simulink model "L_detector_v2"  (Simulink 7.6)
settings: Solver=FixedStepDiscrete  StartTime=0.0  StopTime=0  RelTol=1e-3
values from neighbouring files (symbols this model uses):
  Forward_Camera_Dimensions = [160 120]    [VisionConstants.m]
  Iter_Segment_Thresh = 60    [VisionConstants.m]
undefined symbols (not defined in the file or in its folder): a_range, b_range, Forward_Fov, Rec, SDTV
libraries: vipgeotforms x3, vipconversions x2, viptextngfix x1, vipanalysis x1, viptransforms x1
settings Model: Creator=Thing 1  LastModifiedBy=auvt
settings OptimizationCC: OptimizeModelRefInitCode=on
settings RTWCC: SystemTargetFile=ert.tlc  GenCodeOnly=on  TemplateMakefile=ert_default_tmf  Description=Real-Time Workshop Embedded Coder  GenerateReport=on  ProcessScript=ert_make_rtw_hook  IncludeHyperlinkInReport=on  LaunchReport=on  TargetLang=C++
settings CodeAppCC: IgnoreCustomStorageClasses=off
settings ERTTargetCC: MultiwordLength=2048  GenerateSampleERTMain=on  ERTCustomFileTemplate=example_file_process.tlc  ConvertIfToSwitch=off

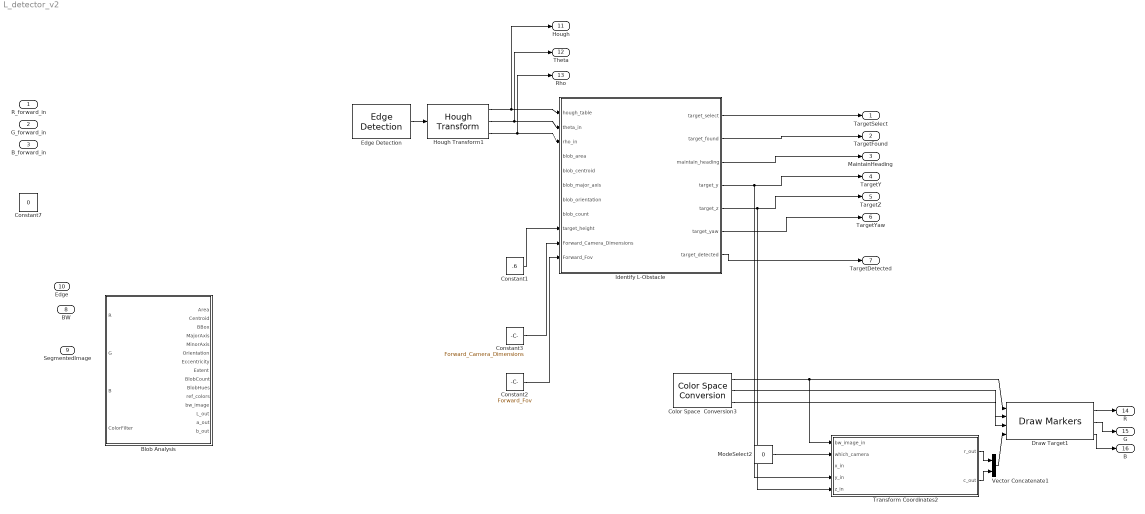
== system L_detector_v2 ==
  R_forward_in : Inport  PortDimensions=Forward_Camera_Dimensions
  G_forward_in : Inport  Port=2  PortDimensions=Forward_Camera_Dimensions
  B_forward_in : Inport  Port=3  PortDimensions=Forward_Camera_Dimensions
  Blob Analysis : Subsystem
  Color Space  Conversion3 : vipconversions/Color Space  Conversion  conversion=Obsolete  conversionActive=L*a*b* to sR'G'B'  wp_str=D50  rec=Rec. 601 (SDTV)  sys=1125/60/2:1  imagePorts=Separate color signals
  Constant1 : Constant  Value=.6  SampleTime=-1
  Constant2 : Constant  Value=Forward_Fov  SampleTime=-1
  Constant3 : Constant  Value=Forward_Camera_Dimensions  SampleTime=-1
  Constant7 : Constant  Value=0  SampleTime=-1
  Draw Target1 : viptextngfix/Draw Markers  DialogController=vipDDGCreate  DialogControllerArgs=DataTag3  shape=X-mark  size=7  fill=off  fillClrSource=Specify via dialog  display=User-specified value  intensity=200  color=[0 0 0]  opacity=0.6  viewport=Entire image  antialiasing=off  inType=Obsolete  imagePorts=Separate color signals  prodOutputMode=Binary point scaling  prodOutputWordLength=32  prodOutputFracLength=14  memoryMode=Specify word length  memoryWordLength=16  memoryFracLength=15  roundingMode=Floor  overflowMode=off
  Edge Detection : vipanalysis/Edge Detection  DialogController=vipDDGCreate  DialogControllerArgs=DataTag4  method=Sobel  outputType=Binary image  userDefinedThreshold=off  thresholdSource=Specify via dialog  threshold=20  thresholdTuning=3  edgeThinning=on  threshold_canny=[0.25 0.60]  autoPercent=70  sigma=1  roundingMode=Floor  overflowMode=off
  Hough Transform1 : viptransforms/Hough Transform  DialogController=vipDDGCreate  DialogControllerArgs=DataTag5  theta_res=pi/180  rho_res=1  out_theta_rho=on  outdtmode=double  firstCoeffMode=Binary point scaling  firstCoeffWordLength=16  firstCoeffFracLength=14  secondCoeffMode=Binary point scaling  secondCoeffWordLength=32  secondCoeffFracLength=16  outputMode=Binary point scaling  outputWordLength=16  outputFracLength=0  accumMode=Binary point scaling  accumWordLength=32  accumFracLength=20  prodOutputMode=Binary point scaling  prodOutputWordLength=32  prodOutputFracLength=20  memoryMode=Binary point scaling  memoryWordLength=32  memoryFracLength=16  roundingMode=Nearest  overflowMode=on
  Identify L-Obstacle : Stateflow chart  TreatAsAtomicUnit=on  SystemSampleTime=[1/30 0]
  ModeSelect2 : Constant  Value=0  SampleTime=-1
  Transform Coordinates2 : Stateflow chart  TreatAsAtomicUnit=on  SystemSampleTime=[1/30 0]
  Vector Concatenate1 : Concatenate  Mode=Multidimensional array
  TargetSelect : Outport  OutDataTypeStr=double
  TargetFound : Outport  Port=2  OutDataTypeStr=double
  MaintainHeading : Outport  Port=3  OutDataTypeStr=double
  TargetY : Outport  Port=4  OutDataTypeStr=double
  TargetZ : Outport  Port=5  OutDataTypeStr=double
  TargetYaw : Outport  Port=6  OutDataTypeStr=double
  TargetDetected : Outport  Port=7  OutDataTypeStr=double
  BW : Outport  Port=8
  SegmentedImage : Outport  Port=9
  Edge : Outport  Port=10
  Hough : Outport  Port=11  OutDataTypeStr=double
  Theta : Outport  Port=12  OutDataTypeStr=double
  Rho : Outport  Port=13  OutDataTypeStr=double
  R : Outport  Port=14  OutDataTypeStr=double
  G : Outport  Port=15  OutDataTypeStr=double
  B : Outport  Port=16  OutDataTypeStr=double
  wires:
  Hough Transform1/1 -> Identify L-Obstacle/1(hough_table), Hough/1
  Hough Transform1/2 -> Identify L-Obstacle/2(theta_in), Theta/1
  Hough Transform1/3 -> Identify L-Obstacle/3(rho_in), Rho/1
  Edge Detection/1 -> Hough Transform1/1
  Identify L-Obstacle/4(target_y) -> TargetY/1, Transform Coordinates2/4(y_in)
  Identify L-Obstacle/5(target_z) -> TargetZ/1, Transform Coordinates2/5(z_in)
  Identify L-Obstacle/7(target_detected) -> TargetDetected/1
  Transform Coordinates2/1(r_out) -> Vector Concatenate1/1
  Transform Coordinates2/2(c_out) -> Vector Concatenate1/2
  Vector Concatenate1/1 -> Draw Target1/4
  ModeSelect2/1 -> Transform Coordinates2/2(which_camera)
  Draw Target1/1 -> R/1
  Draw Target1/2 -> G/1
  Draw Target1/3 -> B/1
  ? -> Edge Detection/1
  ? -> Identify L-Obstacle/4(blob_area)
  ? -> Identify L-Obstacle/5(blob_centroid)
  ? -> Identify L-Obstacle/6(blob_major_axis)
  ? -> Identify L-Obstacle/7(blob_orientation)
  ? -> Identify L-Obstacle/8(blob_count)
  Constant1/1 -> Identify L-Obstacle/9(target_height)
  Identify L-Obstacle/1(target_select) -> TargetSelect/1
  Identify L-Obstacle/2(target_found) -> TargetFound/1
  Identify L-Obstacle/3(maintain_heading) -> MaintainHeading/1
  Identify L-Obstacle/6(target_yaw) -> TargetYaw/1
  Constant3/1 -> Identify L-Obstacle/10(Forward_Camera_Dimensions)
  Constant2/1 -> Identify L-Obstacle/11(Forward_Fov)
  ? -> Color Space  Conversion3/1
  ? -> Color Space  Conversion3/2
  ? -> Color Space  Conversion3/3
  Color Space  Conversion3/1 -> Draw Target1/1, Transform Coordinates2/1(bw_image_in)
  Color Space  Conversion3/2 -> Draw Target1/2
  Color Space  Conversion3/3 -> Draw Target1/3

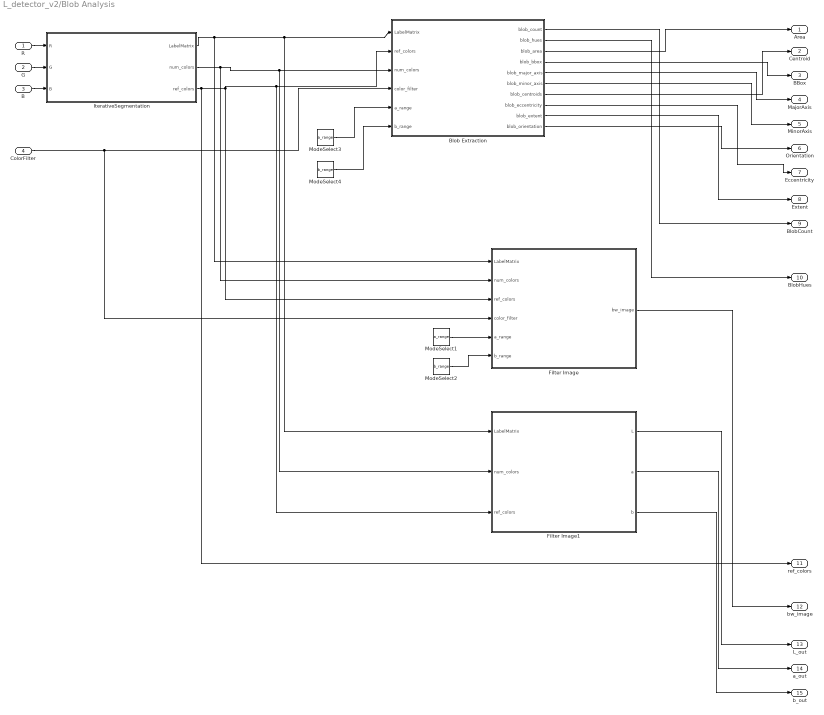
== system L_detector_v2/Blob Analysis ==
  R : Inport
  G : Inport  Port=2
  B : Inport  Port=3
  ColorFilter : Inport  Port=4
  Blob Extraction : Stateflow chart  TreatAsAtomicUnit=on
  Filter Image : Stateflow chart  TreatAsAtomicUnit=on
  Filter Image1 : Stateflow chart  TreatAsAtomicUnit=on
  IterativeSegmentation : Subsystem
      settings: UndoDeleteFcn=Stateflow.SLINSF.SimulinkMan.restorePreDeleteFcn  PreDeleteFcn=Stateflow.SLINSF.SimulinkMan.removePreDeleteFcn
  ModeSelect1 : Constant  Value=a_range  SampleTime=-1
  ModeSelect2 : Constant  Value=b_range  SampleTime=-1
  ModeSelect3 : Constant  Value=a_range  SampleTime=-1
  ModeSelect4 : Constant  Value=b_range  SampleTime=-1
  Area : Outport
  Centroid : Outport  Port=2
  BBox : Outport  Port=3
  MajorAxis : Outport  Port=4
  MinorAxis : Outport  Port=5
  Orientation : Outport  Port=6
  Eccentricity : Outport  Port=7
  Extent : Outport  Port=8
  BlobCount : Outport  Port=9
  BlobHues : Outport  Port=10
  ref_colors : Outport  Port=11
  bw_image : Outport  Port=12
  L_out : Outport  Port=13
  a_out : Outport  Port=14
  b_out : Outport  Port=15
  wires:
  Filter Image1/3(b) -> b_out/1
  Filter Image1/2(a) -> a_out/1
  Filter Image1/1(L) -> L_out/1
  Filter Image/1(bw_image) -> bw_image/1
  Blob Extraction/2(blob_hues) -> BlobHues/1
  Blob Extraction/1(blob_count) -> BlobCount/1
  Blob Extraction/9(blob_extent) -> Extent/1
  Blob Extraction/8(blob_eccentricity) -> Eccentricity/1
  Blob Extraction/10(blob_orientation) -> Orientation/1
  Blob Extraction/6(blob_minor_axis) -> MinorAxis/1
  Blob Extraction/5(blob_major_axis) -> MajorAxis/1
  Blob Extraction/4(blob_bbox) -> BBox/1
  Blob Extraction/7(blob_centroids) -> Centroid/1
  Blob Extraction/3(blob_area) -> Area/1
  ColorFilter/1 -> Filter Image/4(color_filter), Blob Extraction/4(color_filter)
  ModeSelect4/1 -> Blob Extraction/6(b_range)
  ModeSelect3/1 -> Blob Extraction/5(a_range)
  ModeSelect2/1 -> Filter Image/6(b_range)
  ModeSelect1/1 -> Filter Image/5(a_range)
  IterativeSegmentation/3(ref_colors) -> ref_colors/1, Filter Image1/3(ref_colors), Blob Extraction/2(ref_colors), Filter Image/3(ref_colors)
  IterativeSegmentation/2(num_colors) -> Filter Image1/2(num_colors), Blob Extraction/3(num_colors), Filter Image/2(num_colors)
  IterativeSegmentation/1(LabelMatrix) -> Filter Image1/1(LabelMatrix), Blob Extraction/1(LabelMatrix), Filter Image/1(LabelMatrix)
  B/1 -> IterativeSegmentation/3(B)
  G/1 -> IterativeSegmentation/2(G)
  R/1 -> IterativeSegmentation/1(R)

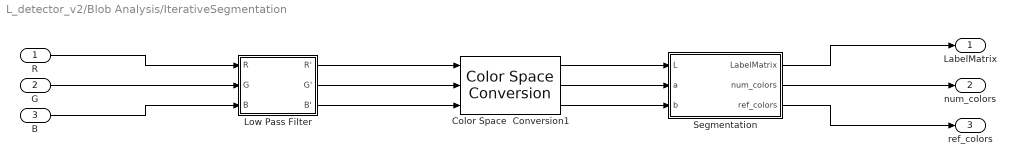
== system L_detector_v2/Blob Analysis/IterativeSegmentation ==
  R : Inport
  G : Inport  Port=2
  B : Inport  Port=3
  Color Space  Conversion1 : vipconversions/Color Space  Conversion  conversion=Obsolete  conversionActive=sR'G'B' to L*a*b*  wp_str=D50  rec=Rec. 601 (SDTV)  sys=1125/60/2:1  imagePorts=Separate color signals
  Low Pass Filter : Subsystem
  Segmentation : Subsystem
  LabelMatrix : Outport
  num_colors : Outport  Port=2
  ref_colors : Outport  Port=3
  wires:
  B/1 -> Low Pass Filter/3(B)
  G/1 -> Low Pass Filter/2(G)
  R/1 -> Low Pass Filter/1(R)
  Color Space  Conversion1/1 -> Segmentation/1(L)
  Color Space  Conversion1/2 -> Segmentation/2(a)
  Color Space  Conversion1/3 -> Segmentation/3(b)
  Low Pass Filter/1(R') -> Color Space  Conversion1/1
  Low Pass Filter/2(G') -> Color Space  Conversion1/2
  Low Pass Filter/3(B') -> Color Space  Conversion1/3
  Segmentation/1(LabelMatrix) -> LabelMatrix/1
  Segmentation/2(num_colors) -> num_colors/1
  Segmentation/3(ref_colors) -> ref_colors/1

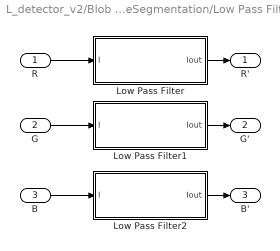
== system L_detector_v2/Blob Analysis/IterativeSegmentation/Low Pass Filter ==
  R : Inport
  G : Inport  Port=2
  B : Inport  Port=3
  Low Pass Filter : Stateflow chart  TreatAsAtomicUnit=on
  Low Pass Filter1 : Stateflow chart  TreatAsAtomicUnit=on
  Low Pass Filter2 : Stateflow chart  TreatAsAtomicUnit=on
  R' : Outport
  G' : Outport  Port=2
  B' : Outport  Port=3
  wires:
  R/1 -> Low Pass Filter/1(I)
  G/1 -> Low Pass Filter1/1(I)
  B/1 -> Low Pass Filter2/1(I)
  Low Pass Filter1/1(Iout) -> G'/1
  Low Pass Filter2/1(Iout) -> B'/1
  Low Pass Filter/1(Iout) -> R'/1

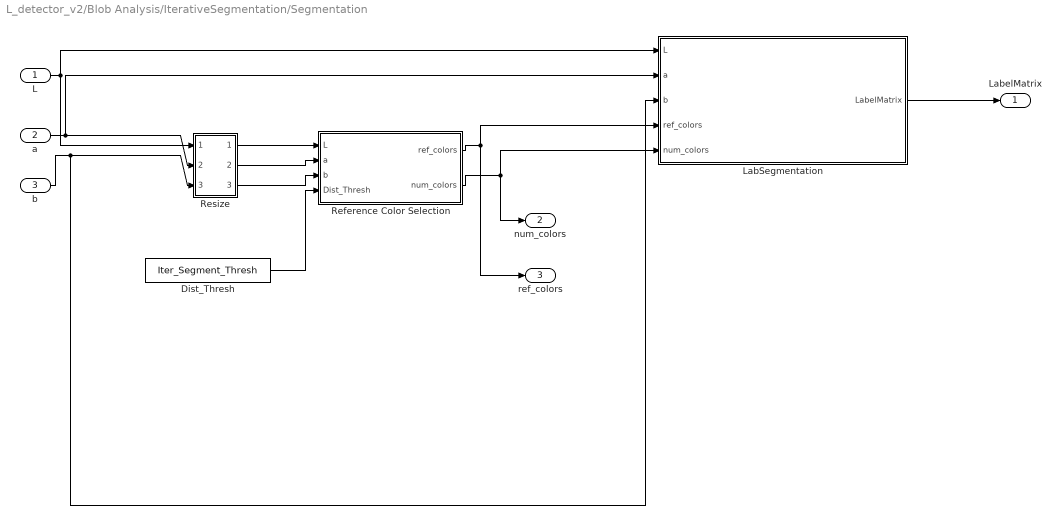
== system L_detector_v2/Blob Analysis/IterativeSegmentation/Segmentation ==
  L : Inport
  a : Inport  Port=2
  b : Inport  Port=3
  Dist_Thresh : Constant  Value=Iter_Segment_Thresh  SampleTime=-1
  LabSegmentation : Stateflow chart  TreatAsAtomicUnit=on
  Reference Color Selection : Stateflow chart  TreatAsAtomicUnit=on
  Resize : Subsystem
  LabelMatrix : Outport
  num_colors : Outport  Port=2
  ref_colors : Outport  Port=3
  wires:
  L/1 -> Resize/1(In1), LabSegmentation/1(L)
  a/1 -> Resize/2(In2), LabSegmentation/2(a)
  b/1 -> Resize/3(In3), LabSegmentation/3(b)
  Resize/1(Out1) -> Reference Color Selection/1(L)
  Resize/2(Out2) -> Reference Color Selection/2(a)
  Resize/3(Out3) -> Reference Color Selection/3(b)
  Reference Color Selection/1(ref_colors) -> LabSegmentation/4(ref_colors), ref_colors/1
  Reference Color Selection/2(num_colors) -> num_colors/1, LabSegmentation/5(num_colors)
  LabSegmentation/1(LabelMatrix) -> LabelMatrix/1
  Dist_Thresh/1 -> Reference Color Selection/4(Dist_Thresh)

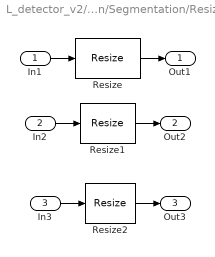
== system L_detector_v2/Blob Analysis/IterativeSegmentation/Segmentation/Resize ==
  In1 : Inport
  In2 : Inport  Port=2
  In3 : Inport  Port=3
  Resize : vipgeotforms/Resize  DialogController=vipDDGCreate  DialogControllerArgs=DataTag0  specify=Number of output rows and columns  rfactor=[]  outCols=25  outRows=25  outRowsCols=[60 80]  interp_method=Bilinear  antialias=on  useROI=off  roiFlag=off  prodOutputMode=Binary point scaling  prodOutputWordLength=32  prodOutputFracLength=10  roundingMode=Nearest  overflowMode=on
  Resize1 : vipgeotforms/Resize  DialogController=vipDDGCreate  DialogControllerArgs=DataTag1  specify=Number of output rows and columns  rfactor=[200 150]  outCols=25  outRows=25  outRowsCols=[60 80]  interp_method=Bilinear  antialias=on  useROI=off  roiFlag=off  prodOutputMode=Binary point scaling  prodOutputWordLength=32  prodOutputFracLength=10  roundingMode=Nearest  overflowMode=on
  Resize2 : vipgeotforms/Resize  DialogController=vipDDGCreate  DialogControllerArgs=DataTag2  specify=Number of output rows and columns  rfactor=[200 150]  outCols=25  outRows=25  outRowsCols=[60 80]  interp_method=Bilinear  antialias=on  useROI=off  roiFlag=off  prodOutputMode=Binary point scaling  prodOutputWordLength=32  prodOutputFracLength=10  roundingMode=Nearest  overflowMode=on
  Out1 : Outport
  Out2 : Outport  Port=2
  Out3 : Outport  Port=3
  wires:
  In1/1 -> Resize/1
  Resize/1 -> Out1/1
  In2/1 -> Resize1/1
  Resize1/1 -> Out2/1
  In3/1 -> Resize2/1
  Resize2/1 -> Out3/1

== matlab function Identify L-Obstacle ==
  data: target_select output double; target_found output double; maintain_heading output double; hough_table input double; target_y output double; target_z output double; target_yaw output double; target_detected output double; theta_in input double; rho_in input double; blob_area input double; blob_centroid input double; blob_major_axis input double; blob_orientation input double; blob_count input double; target_height input double; Forward_Camera_Dimensions input double; Forward_Fov input double
function [target_select, target_found, maintain_heading, target_y, target_z, target_yaw, target_detected] = validation_gate(hough_table, theta_in, rho_in, blob_area, blob_centroid, blob_major_axis, blob_orientation, blob_count, target_height, Forward_Camera_Dimensions, Forward_Fov)
%#eml
%{

1. Iteratively segment image
2. Obtain information about all blobs in image
3. Generate a bw image by filtering colors (thresholding)

3.5. Identify one appropriate horizontal and one appropriate vertical blob

4. Perform edge detection then Hough transform to bw image
5. Identify the most popular lines (any orientation) that are:
     a) Nearly colinear with blobs, and
     b) At approximately 90 degrees from each other

6. Target appropriately

%}




% This function attempts to identfiy the L-shaped obstacle, and returns
%   targeting information, and a true/false target_detected parameter.


% Initialize
target_ratio_v = .3;  % Target position inside the gate (0 to 1; 0 for both is the intersection of the horizontal and vertical sections)
target_ratio_h = .3;

target_select = 1;
target_found = 1;
maintain_heading = 0;
target_y = 0;
target_z = 0;
target_yaw = 0;
target_detected = 0;


% Only the (max_num_lines) with the most votes will be considered as
%   candidates for the gate
max_num_lines = 200;
[rho_length, theta_length] = size(hough_table);
rows = Forward_Camera_Dimensions(1);
cols = Forward_Camera_Dimensions(2);

image_area = rows*cols;
area_thresh = 0.8;  % Ratio of blob area to image area considered to imply the blob is actually background noise

% eps_rho must be at least as big as the gate leg diameter (units of
%   pixels)
eps_rho = .1*max(rows,cols);
% eps_theta is used to distinguish lines as "horizontal" or "vertical";
%   units are radians
eps_theta = 10*pi/180;

% These vectors contain the final two lines that compose the validation gate
rho_gate = zeros(1,2);
theta_gate = zeros(1,2);

% These vectors contain intermediate line information; as lines are
%   eliminated from these vectors, their values are set to zero
% Note that rho_in and theta_in are referred to by hough_table; they do not
%   constitute (rho,theta) pairs without hough_table. rho and theta,
%   however, do constitute (rho,theta) pairs.
rho = zeros(1,max_num_lines);
theta = zeros(1,max_num_lines);


% Identify the most popular max_num_lines lines
i_index = ones(1,max_num_lines);
j_index = ones(1,max_num_lines);

for m = 1:max_num_lines
    
    max_votes = 0;
    for i = 1:rho_length
        for j = 1:theta_length
            if( hough_table(i,j) > max_votes )
                i_index(m) = i;
                j_index(m) = j;
                max_votes = hough_table(i,j);
            end
        end
    end
    
    rho(m) = rho_in(i_index(m));
    theta(m) = theta_in(j_index(m));
    hough_table(i_index(m),j_index(m)) = 0;
    
end


% Correct orientations to vehicle coordinates
for j = 1:blob_count
    % theta_hold:
    %   -is between [-pi/2, +pi/2]
    % blob_orientation:
    %   -is potentially outside this range
    %   -needs to be corrected by pi/2 to get relative heading
    blob_orientation(j) = mod(pi - blob_orientation(j), pi) - pi/2;
end


% Determine the most popular lines which are nearly colinear to blobs
theta_hold = theta;
i_gate = zeros(2,2);  % Indices for line and blob, respectively
for g = 1:2
    
    found = 0;
    for i = 1:max_num_lines
        for j = 1:blob_count
            
            % Search for a match between one blob and one line
            condition1 = abs(theta_hold(i) - blob_orientation(j)) <= eps_theta;
            condition2 = blob_area(j)/image_area <= area_thresh;
            condition3 = theta_hold(i) ~= 1000 && blob_orientation(j) ~= 1000;
            c1 = blob_centroid(2,j);
            r1 = blob_centroid(1,j);
            c2 = rho(i)*cos(theta(i)) - r1 + c1*sin(theta(i));
            r2 = -cot(theta(i))*c2 + rho(i)/sin(theta(i));
            d = sqrt( (c2 - c1)^2 + (r2 - r1)^2 );
            condition4 = d <= eps_rho;
            if(condition1 && condition2 && condition3 && condition4)
                
                if(g == 1)
                    
                    % Determine the first gate element
                    i_gate(1,g) = i;
                    i_gate(2,g) = j;
                    
                else
                    
                    % Assume the first gate element was found correctly;
                    %   check that all other gate elements are at right
                    %   angles to the first
                    if( abs((pi/2) - abs(theta_hold(i) - theta_hold( i_gate(1,1) ))) <= eps_theta)
                        i_gate(1,g) = i;
                        i_gate(2,g) = j;
                    end
                    
                end
                
                theta_hold(i) = 1000;  % Invalid angle; do not want this line to be selected again
                blob_orientation(j) = 1000;
                found = 1;
                break;
            end
            
        end
        
        if(found == 1)
            break;
        end
    end
    
end


if( ~(i_gate(1) == 0 && i_gate(2) == 0) )
    
    % Sort elements of i_gate to place the vertical element in the first
    %   position, horizontal element in second position
    ihold = i_gate(1,1);
    jhold = i_gate(2,1);
    if( abs(theta( i_gate(1,1) )) > abs(theta( i_gate(1,2) )) )
        i_gate(1,1) = i_gate(1,2);
        i_gate(2,1) = i_gate(2,2);

        i_gate(1,2) = ihold;
        i_gate(2,2) = jhold;
    end


    % Assign appropriate gate information
    for g = 1:2
        rho_gate(g) = rho( i_gate(1,g) );
        theta_gate(g) = theta( i_gate(1,g) );
    end


    % Compute targeting information
    % Determine side lengths and distances for target
    length1 = blob_major_axis(i_gate(2,1));
    length2 = blob_major_axis(i_gate(2,2));
    d1 = target_ratio_v*length1;
    d2 = target_ratio_h*length2;

    phi1 = blob_orientation(i_gate(2,1));
    phi2 = blob_orientation(i_gate(2,2));
    theta1 = (pi/2) - phi1;
    theta2 = (pi/2) - phi2;

    r1 = blob_centroid(1,i_gate(2,1));
    c1 = blob_centroid(2,i_gate(2,1));
    r2 = blob_centroid(1,i_gate(2,2));
    c2 = blob_centroid(2,i_gate(2,2));

    rho1 = c1*sin(theta1) + r1*cos(theta1);
    rho2 = c2*sin(theta2) + r2*cos(theta2);

    r3 = (1/( cos(theta1)*sin(theta2) - cos(theta2)*sin(theta1) ))*( rho1*sin(theta2) - rho2*sin(theta1) );
    c3 = -cot(theta1)*r3 + rho1/sin(theta1);
    %r3 = (1/( sin(phi1)*cos(phi2) - sin(phi2)*cos(phi1) ))*( c2 - c1 + sin(pih1)*cos(phi2)*r1 - sin(phi2)*cos(phi1)*r2 );
    %c3 = r3*tan(phi1) + c1 - r1*tan(phi1);

    r4 = r3 - d1*cos(phi1);
    c4 = c3 + d1*sin(phi1);

    r5 = r3 + d2*sin(phi2);
    c5 = c3 + d2*cos(phi2);

    theta4 = theta1;
    theta5 = theta2;

    rho4 = c4*sin(theta4) + r4*cos(theta4);
    rho5 = c5*sin(theta5) + r5*cos(theta5);

    r6 = (1/( cos(theta4)*sin(theta5) - cos(theta5)*sin(theta4) ))*( rho4*sin(theta5) - rho5*sin(theta4) );
    c6 = -cot(theta4)*r6 + rho4/sin(theta4);
    
    target_detected = 1;
    
    % Transform target r, c to global coordinate system
    target_z = r6 - floor(rows/2);
    target_y = c6 - floor(cols/2);
    
    target_yaw = Forward_Fov*( target_y/cols );
    target_detected = 0;
    
else
    
    target_y = 0;
    target_z = 0;
    target_yaw = 0;
    target_detected = 0;
    
end


return

== matlab function Blob Analysis/Blob Extraction ==
  data: LabelMatrix input double; ref_colors input double; num_colors input double; color_filter input double; blob_count output double; blob_hues output double; blob_area output double; blob_bbox output double; blob_major_axis output double; blob_minor_axis output double; blob_centroids output double; blob_eccentricity output double; blob_extent output double; blob_orientation output double; a_range input double; b_range input double
function [blob_count, blob_hues, blob_area, blob_bbox, blob_major_axis, blob_minor_axis, blob_centroids, blob_eccentricity, blob_extent, blob_orientation] = GetBlobInfo(LabelMatrix, ref_colors, num_colors, color_filter, a_range, b_range)

% This function extracts 
% Input
%   

% Initialize
max_num_blobs = 50;
min_blob_area = 5;

[rows, cols] = size(LabelMatrix);
LogicMatrix = false(rows,cols);

blob_count = 0;
blob_hues = zeros(3,max_num_blobs);

blob_area = -1.*ones(1,max_num_blobs);
blob_bbox = zeros(4,max_num_blobs);
blob_major_axis = zeros(1,max_num_blobs);
blob_minor_axis = zeros(1,max_num_blobs);
blob_centroids = zeros(2,max_num_blobs);
blob_eccentricity = zeros(1,max_num_blobs);
blob_extent = zeros(1,max_num_blobs);
blob_orientation = zeros(1,max_num_blobs);


% Input hblob, a matrix containing [Area, blob_centroids, Eccentricity] for each
% identified blob
persistent hblob
if isempty(hblob)
    hblob = video.BlobAnalysis('AreaOutputPort',true,'CentroidOutputPort',true,...
        'BoundingBoxOutputPort',true,'MajorAxisLengthOutputPort',true,'MinorAxisLengthOutputPort',true,...
        'OrientationOutputPort',true,...
        'EccentricityOutputPort',true,'ExtentOutputPort',true,'NumBlobsOutputPort',true,...
        'MinimumBlobAreaSource','Property','MinimumBlobArea', min_blob_area);
end


% Calculate geometric information about the blobs
%
% LogicMatrix is a binary version of LabelMatrix, with ones at all
%   locations for which color values are k, and zeros everywhere else
for k = 1:num_colors

    a = ref_colors(k, 2);
    b = ref_colors(k, 3);

    if( color_filter == 0 )
        condition = 1;
    else
        if( a >= a_range(1,5) && a <= a_range(2,5) && b >= b_range(1,5) && b <= b_range(2,5) )
            condition = 1;
        else
            condition = 0;
        end
    end
    
    if( condition == 1 )
        
        for i = 1:rows
            for j = 1:cols
                if(LabelMatrix(i,j) ~= k)
                    LogicMatrix(i,j) = false;
                else
                    LogicMatrix(i,j) = true;
                end
            end
        end

        [TArea,TCentroid,TBBox,TMajorAxis,TMinorAxis,TOrientation,TEccent,TExtent,TNumBlobs] = step(hblob,LogicMatrix);

        for i = 1:TNumBlobs
            if(blob_count + TNumBlobs <= max_num_blobs)

                blob_centroids(1,blob_count+i) = TCentroid(1,i);
                blob_centroids(2,blob_count+i) = TCentroid(2,i);

                ii = round(blob_centroids(1,blob_count+i));
                jj = round(blob_centroids(2,blob_count+i));

                blob_hues(1,blob_count+i) = ref_colors( LabelMatrix(ii,jj), 1 );
                blob_hues(2,blob_count+i) = ref_colors( LabelMatrix(ii,jj), 2 );
                blob_hues(3,blob_count+i) = ref_colors( LabelMatrix(ii,jj), 3 );

                blob_area(blob_count+i) = TArea(i);
                blob_bbox(blob_count+i) = TBBox(i);
                blob_major_axis(blob_count+i) = TMajorAxis(i);
                blob_minor_axis(blob_count+i) = TMinorAxis(i);
                blob_eccentricity(blob_count+i) = TEccent(i);
                blob_extent(blob_count+i) = TExtent(i);
                blob_orientation(blob_count+i) = TOrientation(i);

            end
        end

        blob_count = blob_count + double(TNumBlobs);

    end
    
end


return

== matlab function Transform Coordinates2 ==
  data: bw_image_in input double; which_camera input double; x_in input double; y_in input double; r_out output double; c_out output double; z_in input double
function [r_out, c_out] = transform_G2L(bw_image_in, which_camera, x_in, y_in, z_in)
% This function, "transform Global to Local coordinates," transforms
%   global coordinates that are sent to the controller into local
%   coordinates that can be displayed over images.
%
% 5-29-11
%
% Input
%   x_in, y_in, z_in = vectors of points in global (vehicle-centered)
%     coordinate system
%   bw_image_in = a 2-D array of pixel values (used only to extract image
%     size)
%   which_camera = selects which camera for relative coordinates
%                = 0 -> Forward camera
%                = 1 -> Down camera
%
% Output
%   r_out, c_out = row, column pairs in local coordinate system

[rows, cols] = size(bw_image_in);
if( which_camera == 0 )
    r_out = z_in + floor(rows/2);
    c_out = y_in + floor(cols/2);
else
    r_out = floor(rows/2) - x_in;
    c_out = y_in + floor(cols/2);
end

return

== matlab function Blob Analysis/Filter Image ==
  data: LabelMatrix input double; num_colors input double; ref_colors input double; color_filter input double; bw_image output double; a_range input double; b_range input double
function bw_image = Filter_Image(LabelMatrix, num_colors, ref_colors, color_filter, a_range, b_range)


% Initialize
[rows,cols] = size(LabelMatrix);
bw_image = zeros(rows,cols);


if( color_filter == 1 )
    
    % Allow only colors in specified range
    for r = 1:rows
        for c = 1:cols

            a = ref_colors(LabelMatrix(r,c), 2);
            b = ref_colors(LabelMatrix(r,c), 3);

            if( a >= a_range(1,5) && a <= a_range(2,5) && b >= b_range(1,5) && b <= b_range(2,5) )
                bw_image(r,c) = 1;
            end

        end
    end
    
else
    
    % Generate a bw image using color indices
    maxValue = max(max(max(LabelMatrix)));
    if(maxValue == 0)
        maxValue = 1;
    end
    for r = 1:rows
        for c = 1:cols
            bw_image(r,c) = LabelMatrix(r,c)/maxValue;
        end
    end
    
end


return

== matlab function Blob Analysis/Filter Image1 ==
  data: LabelMatrix input double; num_colors input double; ref_colors input double; L output double; a output double; b output double
function [L, a, b] = Display_Image(LabelMatrix, num_colors, ref_colors)


% Initialize
[rows,cols] = size(LabelMatrix);
bw_image = zeros(rows,cols);
L = zeros(rows,cols);
a = zeros(rows,cols);
b = zeros(rows,cols);


% Allow only colors in specified range
for r = 1:rows
    for c = 1:cols
        
        L(r,c) = ref_colors(LabelMatrix(r,c), 1);
        a(r,c) = ref_colors(LabelMatrix(r,c), 2);
        b(r,c) = ref_colors(LabelMatrix(r,c), 3);
        
    end
end


return

== matlab function Blob Analysis/IterativeSegmentation/Low Pass Filter/Low Pass Filter ==
  data: I input double; Iout output double
function Iout = GaussianBlurr(I)
% This function calculates the gaussian blur of an intensity image

sigma = sqrt(2);

Grows = 3;    % Gaussian matrix rows
Gcols = 3;    % Gaussian matrix columns

[Irows Icols] = size(I);

Iout = double(zeros(Irows,Icols));

Trows = Irows - Grows + 1;
Tcols = Icols - Gcols + 1;
Itemp = double(zeros(Trows,Tcols));

G = zeros(Grows,Gcols);

FirstRow = ceil(-Grows/2);
LastRow = floor(Grows/2);
FirstCol = ceil(-Gcols/2);
LastCol = floor(Gcols/2);
Gsum = 0;
for i=FirstRow:LastRow
    for j = FirstCol:LastCol
        G(i-FirstRow+1,j-FirstCol+1) = exp(-(j*j+i*i)/(2*sigma*sigma));
        Gsum = Gsum + G(i-FirstRow+1,j-FirstCol+1);
    end
end

G = G./Gsum;

Itemp = conv2(double(I),double(G),'valid');

% reflect boundaries to keep image the same size
% top
Iout((1:LastRow),(LastCol+1:Icols-LastCol)) = Itemp((1:LastRow),(1:Tcols));
% bottom
Iout((Irows-LastRow+1:Irows),(LastCol+1:Icols-LastCol)) = Itemp((Trows-LastRow+1:Trows),(1:Tcols));
% left
Iout((1+LastRow:Irows-LastRow),(1:LastCol)) = Itemp((1:Trows),(1:LastCol));
% right
Iout((1+LastRow:Irows-LastRow),(Icols-LastCol+1:Icols)) = Itemp((1:Trows),(Tcols-LastCol+1:Tcols));
% center
Iout((1+LastRow:Irows-LastRow),(1+LastCol:Icols-LastCol)) = Itemp;
% top left corner
Iout(1:LastRow,1:LastCol) = Itemp(1:LastRow,1:LastCol);
% top right corner
Iout(1:LastRow,Icols-LastCol:Icols) = Itemp(1:LastRow,Tcols-LastCol:Tcols);
% bottom left corner
Iout(Irows-LastRow:Irows,1:LastCol) = Itemp(Trows-LastRow:Trows,1:LastCol);
% bottom right corner
Iout(Irows-LastRow:Irows,Icols-LastCol:Icols) = Itemp(Trows-LastRow:Trows,Tcols-LastCol:Tcols);

return

== matlab function Blob Analysis/IterativeSegmentation/Low Pass Filter/Low Pass Filter1 ==
  data: I input double; Iout output double
function Iout = GaussianBlurr(I)
% This function calculates the gaussian blur of an intensity image

sigma = sqrt(2);

Grows = 3;    % Gaussian matrix rows
Gcols = 3;    % Gaussian matrix columns

[Irows Icols] = size(I);

Iout = double(zeros(Irows,Icols));

Trows = Irows - Grows + 1;
Tcols = Icols - Gcols + 1;
Itemp = double(zeros(Trows,Tcols));

G = zeros(Grows,Gcols);

FirstRow = ceil(-Grows/2);
LastRow = floor(Grows/2);
FirstCol = ceil(-Gcols/2);
LastCol = floor(Gcols/2);
Gsum = 0;
for i=FirstRow:LastRow
    for j = FirstCol:LastCol
        G(i-FirstRow+1,j-FirstCol+1) = exp(-(j*j+i*i)/(2*sigma*sigma));
        Gsum = Gsum + G(i-FirstRow+1,j-FirstCol+1);
    end
end

G = G./Gsum;

Itemp = conv2(double(I),double(G),'valid');

% reflect boundaries to keep image the same size
% top
Iout((1:LastRow),(LastCol+1:Icols-LastCol)) = Itemp((1:LastRow),(1:Tcols));
% bottom
Iout((Irows-LastRow+1:Irows),(LastCol+1:Icols-LastCol)) = Itemp((Trows-LastRow+1:Trows),(1:Tcols));
% left
Iout((1+LastRow:Irows-LastRow),(1:LastCol)) = Itemp((1:Trows),(1:LastCol));
% right
Iout((1+LastRow:Irows-LastRow),(Icols-LastCol+1:Icols)) = Itemp((1:Trows),(Tcols-LastCol+1:Tcols));
% center
Iout((1+LastRow:Irows-LastRow),(1+LastCol:Icols-LastCol)) = Itemp;
% top left corner
Iout(1:LastRow,1:LastCol) = Itemp(1:LastRow,1:LastCol);
% top right corner
Iout(1:LastRow,Icols-LastCol:Icols) = Itemp(1:LastRow,Tcols-LastCol:Tcols);
% bottom left corner
Iout(Irows-LastRow:Irows,1:LastCol) = Itemp(Trows-LastRow:Trows,1:LastCol);
% bottom right corner
Iout(Irows-LastRow:Irows,Icols-LastCol:Icols) = Itemp(Trows-LastRow:Trows,Tcols-LastCol:Tcols);

return

== matlab function Blob Analysis/IterativeSegmentation/Low Pass Filter/Low Pass Filter2 ==
  data: I input double; Iout output double
function Iout = GaussianBlurr(I)
% This function calculates the gaussian blur of an intensity image

sigma = sqrt(2);

Grows = 3;    % Gaussian matrix rows
Gcols = 3;    % Gaussian matrix columns

[Irows Icols] = size(I);

Iout = double(zeros(Irows,Icols));

Trows = Irows - Grows + 1;
Tcols = Icols - Gcols + 1;
Itemp = double(zeros(Trows,Tcols));

G = zeros(Grows,Gcols);

FirstRow = ceil(-Grows/2);
LastRow = floor(Grows/2);
FirstCol = ceil(-Gcols/2);
LastCol = floor(Gcols/2);
Gsum = 0;
for i=FirstRow:LastRow
    for j = FirstCol:LastCol
        G(i-FirstRow+1,j-FirstCol+1) = exp(-(j*j+i*i)/(2*sigma*sigma));
        Gsum = Gsum + G(i-FirstRow+1,j-FirstCol+1);
    end
end

G = G./Gsum;

Itemp = conv2(double(I),double(G),'valid');

% reflect boundaries to keep image the same size
% top
Iout((1:LastRow),(LastCol+1:Icols-LastCol)) = Itemp((1:LastRow),(1:Tcols));
% bottom
Iout((Irows-LastRow+1:Irows),(LastCol+1:Icols-LastCol)) = Itemp((Trows-LastRow+1:Trows),(1:Tcols));
% left
Iout((1+LastRow:Irows-LastRow),(1:LastCol)) = Itemp((1:Trows),(1:LastCol));
% right
Iout((1+LastRow:Irows-LastRow),(Icols-LastCol+1:Icols)) = Itemp((1:Trows),(Tcols-LastCol+1:Tcols));
% center
Iout((1+LastRow:Irows-LastRow),(1+LastCol:Icols-LastCol)) = Itemp;
% top left corner
Iout(1:LastRow,1:LastCol) = Itemp(1:LastRow,1:LastCol);
% top right corner
Iout(1:LastRow,Icols-LastCol:Icols) = Itemp(1:LastRow,Tcols-LastCol:Tcols);
% bottom left corner
Iout(Irows-LastRow:Irows,1:LastCol) = Itemp(Trows-LastRow:Trows,1:LastCol);
% bottom right corner
Iout(Irows-LastRow:Irows,Icols-LastCol:Icols) = Itemp(Trows-LastRow:Trows,Tcols-LastCol:Tcols);

return

== matlab function Blob Analysis/IterativeSegmentation/Segmentation/LabSegmentation ==
  data: L input double; LabelMatrix output double; a input double; b input double; ref_colors input double; num_colors input double
function LabelMatrix  = LabSegmentation(L,a,b,ref_colors,num_colors)
% This function generates the label matrix

[rows cols] = size(L);

Lout = zeros(rows,cols);
aout = zeros(rows,cols);
bout = zeros(rows,cols);

LabelMatrix = zeros(rows,cols);

for i = 1:rows
    for j = 1:cols
        min_dist = 1000;
        index = 1;
        for k = 1:num_colors
            dist = sqrt((ref_colors(k,1) - L(i,j))^2 + (ref_colors(k,2) - a(i,j))^2 + (ref_colors(k,3) - b(i,j))^2);
            if(dist < min_dist)
                min_dist = double(dist);
                index = k;
            end
        end
        LabelMatrix(i,j) = index;
    end
end

for i = 1:rows
    for j = 1:cols
        Lout(i,j) = ref_colors(LabelMatrix(i,j),1);
        aout(i,j) = ref_colors(LabelMatrix(i,j),2);
        bout(i,j) = ref_colors(LabelMatrix(i,j),3);
    end
end

cow = 1;

return

== matlab function Blob Analysis/IterativeSegmentation/Segmentation/Reference Color Selection ==
  data: L input double; ref_colors output double; a input double; b input double; num_colors output double; Dist_Thresh input double
function [ref_colors, num_colors] = Segmentation(L,a,b,Dist_Thresh)
% This function tries segmentation by adding new reference colors everytime
% a pixel is found with a distance greater than a certain amount from
% every other reference color

[rows cols] = size(L);

Dist_Threshold = Dist_Thresh;% L = 0 to 100, a = -100 to 100, b = -100 to 100
                    % max dist = 300 -> 60/300 is 20%
x = 1;  % coefficients determining distance calculation
y = 1.5;
z = 1.5;

max_num_colors = 50;
ref_colors = zeros(max_num_colors,3);   % At most 50 different reference colors
LabelMatrix = zeros(rows,cols);
num_colors = 1;

center_row = floor(rows/2);
center_col = floor(cols/2);

% Define first reference color to be colr
ref_colors(1,:) = [L(center_row,center_col) a(center_row,center_col) b(center_row,center_col)];

flag = 0;
i = 1;
j = 1;
while(i <= rows)        % perform initial segmentation
    while(i <= rows && flag == 0)
        while(j <= cols && flag == 0)
            k = 1;
            min_dist = 1000;
            index = 1;
            while(k <= num_colors)
                dist = sqrt(x*(ref_colors(k,1) - L(i,j))^2 + y*(ref_colors(k,2) - a(i,j))^2 + z*(ref_colors(k,3) - b(i,j))^2);
                if(min_dist > dist)
                    min_dist = double(dist);
                    index = k;
                end
                k = k + 1;
            end
            if(j == 117)
                cow = 1;
            end
            if(min_dist > Dist_Threshold && num_colors < max_num_colors)
                ref_colors(num_colors+1,:) = [L(i,j) a(i,j) b(i,j)];
                num_colors = num_colors + 1;
                flag = 1;
                i = 0;
                j = 0;
            else
                LabelMatrix(i,j) = index;
            end
            j = j + 1;
        end
        j = 1;
        i = i + 1;
    end
    flag = 0;
end

% Go through image once more to get more accurate values for the different regions
ref_color_L_avg = zeros(50,1);
ref_color_a_avg = zeros(50,1);
ref_color_b_avg = zeros(50,1);
color_count = zeros(50,1);
for i = 1:rows
    for j = 1:cols
        index = LabelMatrix(i,j);
        ref_color_L_avg(index) = ref_color_L_avg(index) + L(i,j);
        ref_color_a_avg(index) = ref_color_a_avg(index) + a(i,j);
        ref_color_b_avg(index) = ref_color_b_avg(index) + b(i,j);
        color_count(index) = color_count(index) + 1;
    end
end
ref_color_L_avg = ref_color_L_avg ./ color_count;
ref_color_a_avg = ref_color_a_avg ./ color_count;
ref_color_b_avg = ref_color_b_avg ./ color_count;

for i = 1:num_colors
    ref_colors(i,1) = ref_color_L_avg(i);
    ref_colors(i,2) = ref_color_a_avg(i);
    ref_colors(i,3) = ref_color_b_avg(i);
end

return
